simulink model "M_iHGP"  (R2019a)
settings: Solver=VariableStepAuto  StartTime=0.0  StopTime=10.0  RelTol=1e-3
undefined symbols (not defined in the file): ILC_B, M_iinfHGP_aD, M_iinfHGP_bD, M_iinfHGP_cD, M_iinfHGP_dD
settings Model: Creator=jcp2  LastModifiedBy=rache

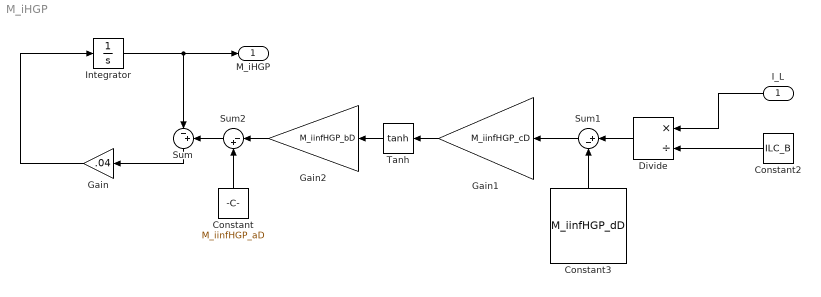
== system M_iHGP ==
  I_L : Inport
  Constant : Constant  Value=M_iinfHGP_aD
  Constant2 : Constant  Value=ILC_B
  Constant3 : Constant  Value=M_iinfHGP_dD
  Divide : Product  Inputs=*/
  Gain : Gain  Gain=.04
  Gain1 : Gain  Gain=M_iinfHGP_cD
  Gain2 : Gain  Gain=M_iinfHGP_bD
  Integrator : Integrator
  Sum : Sum  Inputs=|-+
  Sum1 : Sum  Inputs=|+-
  Sum2 : Sum  Inputs=|-+
  Tanh : Trigonometry  Operator=tanh
  M_iHGP : Outport
  wires:
  Integrator/1 -> Sum/1, M_iHGP/1
  Sum/1 -> Gain/1
  Gain/1 -> Integrator/1
  I_L/1 -> Divide/1
  Constant2/1 -> Divide/2
  Divide/1 -> Sum1/1
  Constant3/1 -> Sum1/2
  Sum1/1 -> Gain1/1
  Gain1/1 -> Tanh/1
  Tanh/1 -> Gain2/1
  Gain2/1 -> Sum2/1
  Constant/1 -> Sum2/2
  Sum2/1 -> Sum/2
